simulink model "Edison_com_reciever"  (R2014a)
settings: Solver=ode45  StartTime=0.0  StopTime=inf  RelTol=1e-3
libraries: amg_usbconverter_n_connect_lib x2
settings Model: Creator=utya  LastModifiedBy=g.kalach

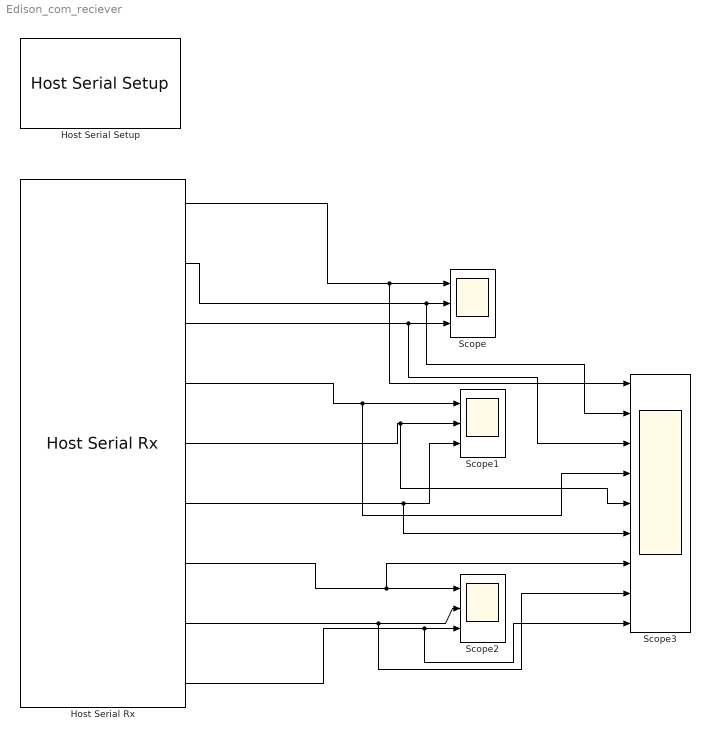
== system Edison_com_reciever ==
  Host Serial Rx : amg_usbconverter_n_connect_lib/Host Serial Rx  conf=rx  port=<auto>  baudrate=115200  databits=8  parity=None  stopbit=1  flowcontrol=None  transfer=Blocking  timeout=5  packetmode=Ascii  enableinitialvalues=off  initialvalues=[]  binheader='7E 7E'  binterminator='03 03'  porttype_double=0  porttype_single=3  porttype_int8=0  porttype_uint8=0  porttype_int16=0  porttype_uint16=0  porttype_int32=0  porttype_uint32=0  asciiformat='%f,%f,%f,%f,%f,%f,%f,%f,%f'  rx_asciiterminator="CRLF (0x0D 0x0A - \"\\r\\n\")"  tx_asciiterminator="CRLF (0x0D 0x0A - \"\\r\\n\")"  sampletime=-1  enablecustomportlabel=off  cinputportlabel=0  coutputportlabel=A  portpinstr=0  blockid=HostSerialRx  inputporttype=[]  inputportwidth=[]  inputportlabel={}  outputporttype=[1 1 1 1 1 1 1 1 1]  outputportwidth=[1 1 1 1 1 1 1 1 1]  outputportlabel={'(single) %f','(single) %f','(single) %f','(single) %f','(single) %f','(single) %f','(single) %f','(single) %f','(single) %f'}  compat=0  optionstring=[]  autoport='COM4'
  Host Serial Setup : amg_usbconverter_n_connect_lib/Host Serial Setup  conf=setup  port=<auto>  baudrate=115200  databits=8  parity=None  stopbit=1  flowcontrol=None  transfer=Blocking  timeout=2  packetmode=Binary  initialvalues=[]  binheader='7E 7E'  binterminator='03 03'  porttype_double=0  porttype_single=1  porttype_int8=0  porttype_uint8=0  porttype_int16=0  porttype_uint16=0  porttype_int32=0  porttype_uint32=2  asciiformat='%d %u %x'  rx_asciiterminator="CRLF (0x0D 0x0A - \"\\r\\n\")"  tx_asciiterminator="CRLF (0x0D 0x0A - \"\\r\\n\")"  sampletime=inf  enablecustomportlabel=off  cinputportlabel=0  coutputportlabel=A  portpinstr=0  blockid=HostSerialSetup  inputporttype=[]  inputportwidth=[]  inputportlabel={}  outputporttype=[]  outputportwidth=[]  outputportlabel={}  compat=0  optionstring=[]  autoport='COM4'
  Scope : Scope  NumInputPorts=3
      settings: TimeRange=1000  YMin=-55~-250~-35  YMax=30~250~45
  Scope1 : Scope  NumInputPorts=3
      settings: TimeRange=1000  YMin=-9000~-9000~-9000  YMax=9000~8000~10000
  Scope2 : Scope  NumInputPorts=3
      settings: TimeRange=1000  YMin=-800~-175~-500  YMax=500~400~550  SaveName=ScopeData2
  Scope3 : Scope  NumInputPorts=9
      settings: TimeRange=1000  YMin=-150~-300~-200~-20000~-20000~-10000~-600~-500~-500  YMax=250~300~250~20000~15000~25000~500~400~400  SaveName=ScopeData3
  wires:
  Host Serial Rx/2 -> Scope3/2, Scope/2
  Host Serial Rx/3 -> Scope3/3, Scope/3
  Host Serial Rx/1 -> Scope3/1, Scope/1
  Host Serial Rx/5 -> Scope3/5, Scope1/2
  Host Serial Rx/4 -> Scope3/4, Scope1/1
  Host Serial Rx/6 -> Scope3/6, Scope1/3
  Host Serial Rx/8 -> Scope3/8, Scope2/2
  Host Serial Rx/7 -> Scope3/7, Scope2/1
  Host Serial Rx/9 -> Scope3/9, Scope2/3
